simulink model "Simulation"  (R2024b)
settings: Solver=FixedStepAuto  StartTime=0.0  StopTime=inf  FixedStep=0.025  RelTol=1e-3
model workspace (MAT data in the model file):
  Ix = 1
  Ixy = 0
  Ixz = 0
  Iy = 1
  Iyx = 0
  Iyz = 0
  Iz = 1
  Izx = 0
  Izy = 0
  Kpd = 0
  Kqd = 0
  Krd = 0
  Kud = 0
  Kvd = 0
  Kwd = 0
  Mpd = 0
  Mqd = 0
  Mrd = 0
  Mud = 0
  Mvd = 0
  Mwd = 0
  Npd = 0
  Nqd = 0
  Nrd = 0
  Nud = 0
  Nvd = 0
  Nwd = 0
  Xpd = 0
  Xqd = 0
  Xrd = 0
  Xud = 0
  Xvd = 0
  Xwd = 0
  Ypd = 0
  Yqd = 0
  Yrd = 0
  Yud = 0
  Yvd = 0
  Ywd = 0
  Zpd = 0
  Zqd = 0
  Zrd = 0
  Zud = 0
  Zvd = 0
  Zwd = 0
  m = 35
  xg = 0
  yg = 0
  zg = 0
values from neighbouring files (symbols this model uses):
  force_values = force_values * 9.81    [initialize_data.m]    (also in matlab.mat = [-22.6611 -28.449 -34.5312 -39.9267 -45.0279 -49.4424 -22.56; vars.mat = [-22.6611 -28.449 -34.5312 -39.9267 -45.0279 -49.4424 -22.56)
  g = 9.81    [matlab.mat]    (also in vars.mat)
  pwm_values = unique(data(:, 2))    [initialize_data.m]    (also in matlab.mat = [1100 1104 1108 1112 1116 1120 1124 1128 1132 1136 1140 1144; vars.mat = [1100 1104 1108 1112 1116 1120 1124 1128 1132 1136 1140 1144)
  rho = 1000    [matlab.mat]
  thruster_dir = [0.5 0 0 0.5 0.5 0 0 0.5 -0.5 0 0 -0.5 ... (24 elements, 8x3)]    [matlab.mat]    (also in vars.mat)
  thruster_pos = [0.218 -0.218 -0.218 0.218 0.36 -0.36 -0.36 0.36 0.25 0.25 -0.25 -0.25 ... (24 elements, 8x3)]    [matlab.mat]    (also in vars.mat)
  V = 0.05061242    [matlab.mat]
  voltage_values = unique(data(:, 1))    [initialize_data.m]    (also in matlab.mat = [10 12 14 16 18 20]; vars.mat = [10 12 14 16 18 20])
libraries: sim3dlib x3, mssSimulink x1, ros2lib x1
settings Model: Creator=elite  LastModifiedBy=user

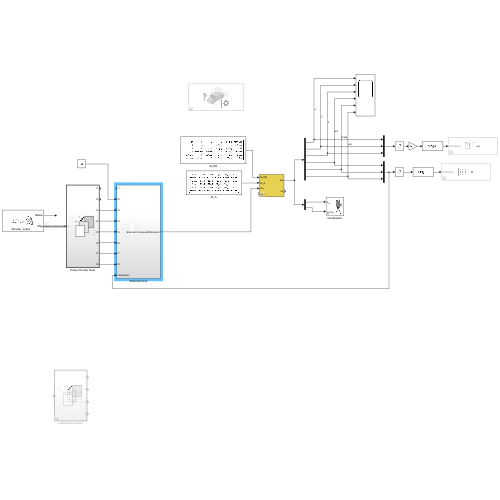
[thumbnail: Simulink's stored preview of the top-level diagram]
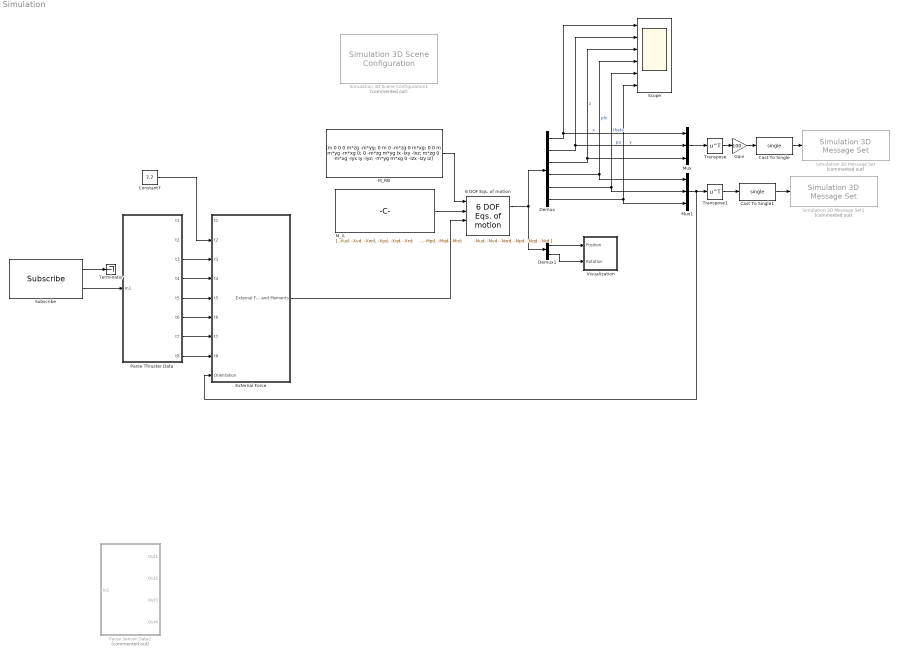
== system Simulation ==
  6 DOF Eqs. of motion : mssSimulink/Modelling/Kinetics /6 DOF Eqs. of motion  CoriolisOnOff=on  nu0=[0 0 0 0 0 0]  eta0=[0 0 0 0 0 0]
  Cast To Single : DataTypeConversion  OutDataTypeStr=single  SaturateOnIntegerOverflow=off  RndMeth=Floor
  Cast To Single1 : DataTypeConversion  OutDataTypeStr=single  SaturateOnIntegerOverflow=off  RndMeth=Floor
  Constant7 : Constant  Value=7.7
  Demux : Demux  Outputs=6
  Demux1 : Demux  Outputs=2
  External Force : Subsystem
  Gain : Gain  Gain=100
  M_A : Constant  Value=|  VectorParams1D=off
      | [ -Xud, -Xvd, -Xwd, -Xpd, -Xqd, -Xrd;
      |         -Yud, -Yvd, -Ywd, -Ypd, -Yqd, -Yrd;
      |         -Zud, -Zvd, -Zwd, -Zpd, -Zqd, -Zrd;
      |         -Kud, -Kvd, -Kwd, -Kpd, -Kqd, -Krd;
      |         -Mud, -Mvd, -Mwd, -Mpd, -Mqd, -Mrd;
      |         -Nud, -Nvd, -Nwd, -Npd, -Nqd, -Nrd ]
  M_RB : Constant  Value=|  VectorParams1D=off
      | [m 0 0 0 m*zg -m*yg; 
      |  0 m 0 -m*zg 0 m*xg; 
      |  0 0 m m*yg -m*xg 0; 
      |  0 -m*zg m*yg Ix -Ixy -Ixz; 
      |  m*zg 0 -m*xg -Iyx Iy -Iyz; 
      |  -m*yg m*xg 0 -Izx -Izy Iz]
  Mux : Mux  Inputs=3
  Mux1 : Mux  Inputs=3
  Parse Sensor Data1 : Subsystem  Commented=on  TreatAsAtomicUnit=on
  Parse Thruster Data : Subsystem  TreatAsAtomicUnit=on
  Scope : Scope  NumInputPorts=6
  Simulation 3D Message Set : sim3dlib/Simulation 3D Message Set  Priority=-1  Commented=on  SigName=pos  Ts=-1  aMode=2
      settings: LibrarySourceBlock=vehdynlibsim3dcore/Simulation 3D Message Set
  Simulation 3D Message Set1 : sim3dlib/Simulation 3D Message Set  Priority=-1  Commented=on  SigName=rot  Ts=-1  aMode=2
      settings: LibrarySourceBlock=vehdynlibsim3dcore/Simulation 3D Message Set
  Simulation 3D Scene Configuration1 : sim3dlib/Simulation 3D Scene Configuration  Priority=0  Commented=on  ProjectFormat=Unreal Editor  SceneDesc=Empty scene  ProjectName=C:\Program Files\MATLAB\R2024b\toolbox\shared\sim3d_projects\automotive_project_windows\UE\WindowsNoEditor\VehicleSimulation.exe  ScenePath=/Game/Maps/HwStrght  UEProjPath=C:\Users\user\Desktop\RoboSub MSDP\AUV_Visualization\AUV_Visualization.uproject  EnableOpenDRIVE=off  vehTagList={'Custom';'Scene Origin'}  vehTag=Scene Origin  FreeCameraInitialTranslation=[0, 0, 0]  FreeCameraDefaultInitialTranslation=[-6, 0, 2]  FreeCameraInitialRotation=[0, 0, 0]  FreeCameraDefaultInitialRotation=[0, -15, 0]  OpVisEn=off  Ts=0.025  EnableWindow=on  EnableRemoteAccess=off  EnableWeather=off  SunAzimuth=90  SunAltitude=40.0  EnableGeospatialSun=off  Latitude=0  Longitude=0  Date=2023-01-01  Time=10:30:00  GeoTimeZone=-5.0  SunDaylightSaving=off  wind=1  clouds=10  EnableVolumetricClouds=off  CloudCoverage=0  CloudAltitude=6  fog=0  rain=0  RaindropsEffect=off  SnowDensity=0  EnableGeospatial=off  UseTrueOrigin=off  OriginHeight=200  OriginLatitude=40.744652  OriginLongitude=-73.988864  MapStyle=Aerial  AdditionalAssetIDs=[]  UseAdvancedSunSky=off  SolarTime=11  TimeZone=-5  Day=21  Month=9  Year=2022  UseDaylightSavingTime=on  DSTStartDay=10  DSTStartMonth=3  DSTEndDay=3  DSTEndMonth=11  DSTSwitchHour=2  sensorTag=MainCamera2  sensorId=2  sensorName=MainCamera2  mountLoc=Origin  offsetFlag=off  tmountOffset=[0, 0, 0]  rmountOffset=[0, 0, 0]  HorizontalResolution=1280  VerticalResolution=720  HorizontalFOV=60  mountPoint=[0 0 0]  mountOrientation=[0 0 0]  aMode=5  ID=2  GeoTrigger=Inactive
      settings: LibrarySourceBlock=sl3dlib/Simulation 3D/Environment/Simulation 3D Scene Configuration
  Subscribe : ros2lib/Subscribe  topicSource=Select from ROS network  topic=/thruster_output  messageType=std_msgs/String  sampleTime=-1  QOSHistory=Keep last  QOSDepth=1  QOSReliability=Reliable  QOSDurability=Volatile  QOSDeadline=Inf  QOSLifespan=Inf  QOSLiveliness=Automatic  QOSLeaseDuration=Inf  QOSAvoidROSNamespaceConventions=off
  Terminator : Terminator
  Transpose : Math  Operator=transpose
  Transpose1 : Math  Operator=transpose
  Visualization : Subsystem  mask(6DoF_Animation){u2=0.1, u8=on}
      mask prompts: u2 "aeroblks:aeroblkanim6dof:block6DoF_AnimationParamTimeintervalbetweenupdates"; u8 "aeroblks:aeroblkanim6dof:block6DoF_AnimationParamEnableanimation"
      mask help: aeroblks:aeroblkanim6dof:block6DoF_AnimationDesc
      mask init:
      | aeroicon('aeroblk');
      | Config.update = u2;
      | Config.Animenable = u8;
      | Config.Model = bdroot(gcb);
      mask Help: eval('asbhelp(''sixdof_animation'')');
      mask DialogControl DescGroupVar Prompt: Animation
      mask DialogControl DescTextVar Prompt: Show animation of body
      mask DialogControl u2 Prompt: Time interval between updates:
      mask DialogControl u8 Prompt: Enable animation
      mask Display:
      | port_label('input',1,'x_e','texmode','on');
      | port_label('input',2,'\phi \theta \psi','texmode','on');
  wires:
  M_RB/1 -> 6 DOF Eqs. of motion/1
  M_A/1 -> 6 DOF Eqs. of motion/2
  6 DOF Eqs. of motion/1 -> Demux/1, Demux1/1
  Demux/1 -> Mux/1, Scope/1  "x"
  Demux/2 -> Mux/2, Scope/2  "y"
  Demux/4 -> Scope/4, Mux1/1  "phi"
  Demux/5 -> Scope/5, Mux1/2  "theta"
  Demux/6 -> Scope/6, Mux1/3  "psi"
  Demux/3 -> Mux/3, Scope/3  "z"
  Demux1/1 -> Visualization/1(Position)
  Demux1/2 -> Visualization/2(Rotation)
  Subscribe/2 -> Parse Thruster Data/1(In1)
  Subscribe/1 -> Terminator/1
  Mux1/1 -> External Force/9(Orientation), Transpose1/1
  Mux/1 -> Transpose/1
  Transpose/1 -> Gain/1
  Gain/1 -> Cast To Single/1
  Cast To Single/1 -> Simulation 3D Message Set/1
  Transpose1/1 -> Cast To Single1/1
  Cast To Single1/1 -> Simulation 3D Message Set1/1
  Constant7/1 -> External Force/2(t2)
  Parse Thruster Data/3(t3) -> External Force/3(t3)
  Parse Thruster Data/4(t4) -> External Force/4(t4)
  Parse Thruster Data/5(t5) -> External Force/5(t5)
  Parse Thruster Data/6(t6) -> External Force/6(t6)
  Parse Thruster Data/7(t7) -> External Force/7(t7)
  Parse Thruster Data/8(t8) -> External Force/8(t8)
  External Force/1(External Forces and Moments) -> 6 DOF Eqs. of motion/3

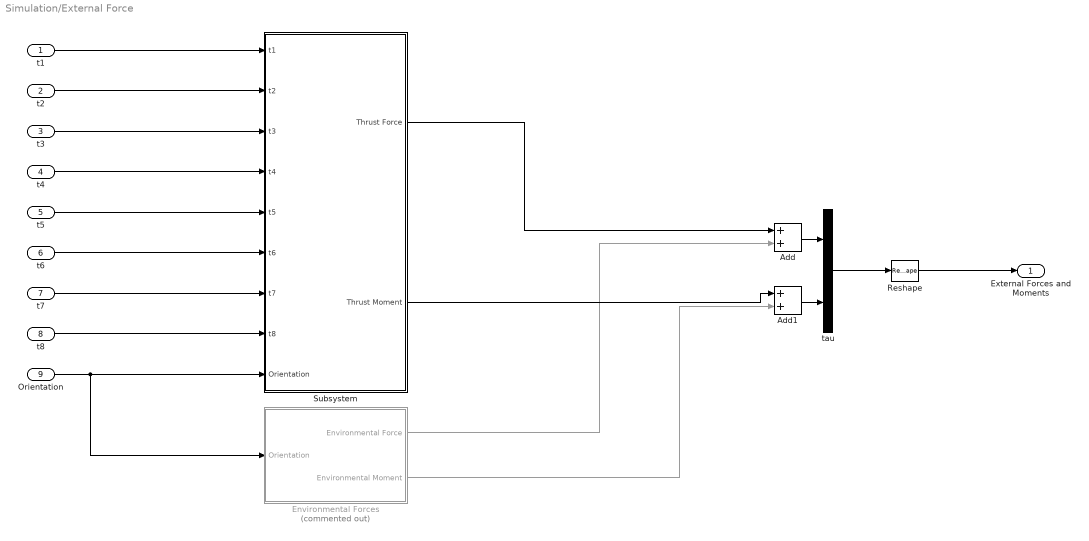
== system Simulation/External Force ==
  t1 : Inport
  t2 : Inport  Port=2
  t3 : Inport  Port=3
  t4 : Inport  Port=4
  t5 : Inport  Port=5
  t6 : Inport  Port=6
  t7 : Inport  Port=7
  t8 : Inport  Port=8
  Orientation : Inport  Port=9
  Add : Sum
  Add1 : Sum
  Environmental Forces : Subsystem  Commented=on
  Reshape : Reshape
  Subsystem : Subsystem
  tau : Mux  Inputs=2
  External Forces and Moments : Outport
  wires:
  tau/1 -> Reshape/1
  Reshape/1 -> External Forces and Moments/1
  Environmental Forces/1(Environmental Force) -> Add/2
  t1/1 -> Subsystem/1(t1)
  t2/1 -> Subsystem/2(t2)
  t3/1 -> Subsystem/3(t3)
  t4/1 -> Subsystem/4(t4)
  t5/1 -> Subsystem/5(t5)
  t6/1 -> Subsystem/6(t6)
  t7/1 -> Subsystem/7(t7)
  t8/1 -> Subsystem/8(t8)
  Orientation/1 -> Environmental Forces/1(Orientation), Subsystem/9(Orientation)
  Subsystem/1(Thrust Force) -> Add/1
  Add/1 -> tau/1
  Add1/1 -> tau/2
  Subsystem/2(Thrust Moment) -> Add1/1
  Environmental Forces/2(Environmental Moment) -> Add1/2

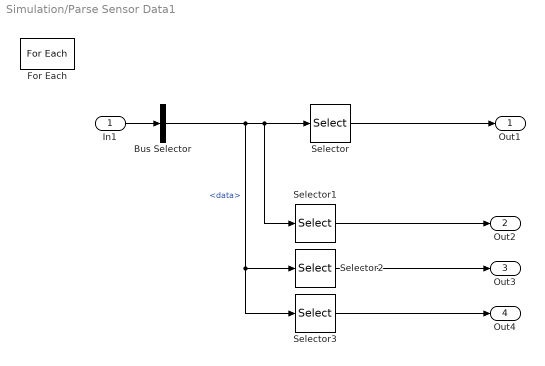
== system Simulation/Parse Sensor Data1 ==
  In1 : Inport  Partition=on  PartitionDimension=1  PartitionWidth=1  PartitionOffset=0
  Bus Selector : BusSelector  OutputSignals=data
  For Each : ForEach  DisableCoverage=on
  Selector : Selector  InputPortWidth=128  IndexOptions=Index vector (dialog)  Indices=1  OutputSizes=1
  Selector1 : Selector  InputPortWidth=128  IndexOptions=Index vector (dialog)  Indices=2  OutputSizes=1
  Selector2 : Selector  InputPortWidth=128  IndexOptions=Index vector (dialog)  Indices=3  OutputSizes=1
  Selector3 : Selector  InputPortWidth=128  IndexOptions=Index vector (dialog)  Indices=4  OutputSizes=1
  Out1 : Outport  ConcatenationDimension=1
  Out2 : Outport  Port=2  ConcatenationDimension=1
  Out3 : Outport  Port=3  ConcatenationDimension=1
  Out4 : Outport  Port=4  ConcatenationDimension=1
  wires:
  In1/1 -> Bus Selector/1
  Selector3/1 -> Out4/1
  Selector/1 -> Out1/1
  Selector2/1 -> Out3/1
  Selector1/1 -> Out2/1
  Bus Selector/1 -> Selector/1, Selector1/1, Selector3/1, Selector2/1  "<data>"

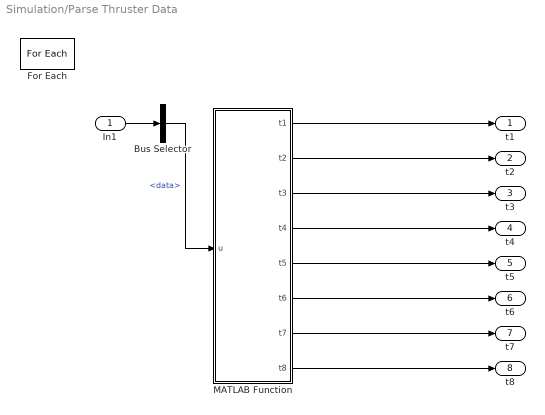
== system Simulation/Parse Thruster Data ==
  In1 : Inport  Partition=on  PartitionDimension=1  PartitionWidth=1  PartitionOffset=0
  Bus Selector : BusSelector  OutputSignals=data
  For Each : ForEach  DisableCoverage=on
  MATLAB Function : MATLAB Function  TreatAsAtomicUnit=on
  t1 : Outport  ConcatenationDimension=1
  t2 : Outport  Port=2  ConcatenationDimension=1
  t3 : Outport  Port=3  ConcatenationDimension=1
  t4 : Outport  Port=4  ConcatenationDimension=1
  t5 : Outport  Port=5  ConcatenationDimension=1
  t6 : Outport  Port=6  ConcatenationDimension=1
  t7 : Outport  Port=7  ConcatenationDimension=1
  t8 : Outport  Port=8  ConcatenationDimension=1
  wires:
  In1/1 -> Bus Selector/1
  MATLAB Function/4(t4) -> t4/1
  MATLAB Function/1(t1) -> t1/1
  MATLAB Function/3(t3) -> t3/1
  MATLAB Function/2(t2) -> t2/1
  Bus Selector/1 -> MATLAB Function/1(u)  "<data>"
  MATLAB Function/5(t5) -> t5/1
  MATLAB Function/6(t6) -> t6/1
  MATLAB Function/7(t7) -> t7/1
  MATLAB Function/8(t8) -> t8/1

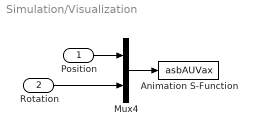
== system Simulation/Visualization ==
  Position : Inport
  Rotation : Inport  Port=2  Unit=rad
  Animation S-Function : M-S-Function  FunctionName=asbAUVax  Parameters=Config
  Mux4 : Mux  Inputs=2
  wires:
  Rotation/1 -> Mux4/2
  Mux4/1 -> Animation S-Function/1
  Position/1 -> Mux4/1

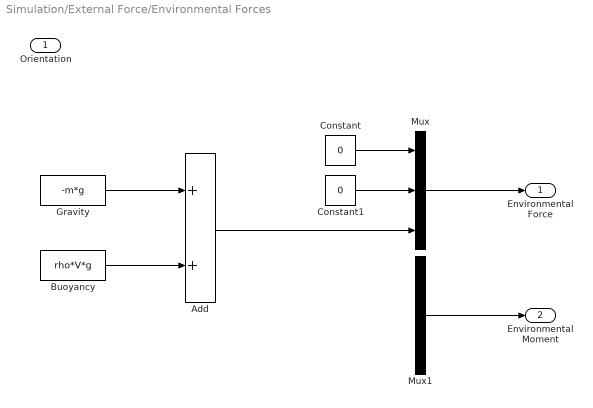
== system Simulation/External Force/Environmental Forces ==
  Orientation : Inport
  Add : Sum
  Buoyancy : Constant  Value=rho*V*g
  Constant : Constant  Value=0
  Constant1 : Constant  Value=0
  Gravity : Constant  Value=-m*g
  Mux : Mux  Inputs=3
  Mux1 : Mux  Inputs=3
  Environmental Force : Outport
  Environmental Moment : Outport  Port=2
  wires:
  Buoyancy/1 -> Add/2
  Gravity/1 -> Add/1
  Mux/1 -> Environmental Force/1
  Add/1 -> Mux/3
  Constant/1 -> Mux/1
  Constant1/1 -> Mux/2
  Mux1/1 -> Environmental Moment/1

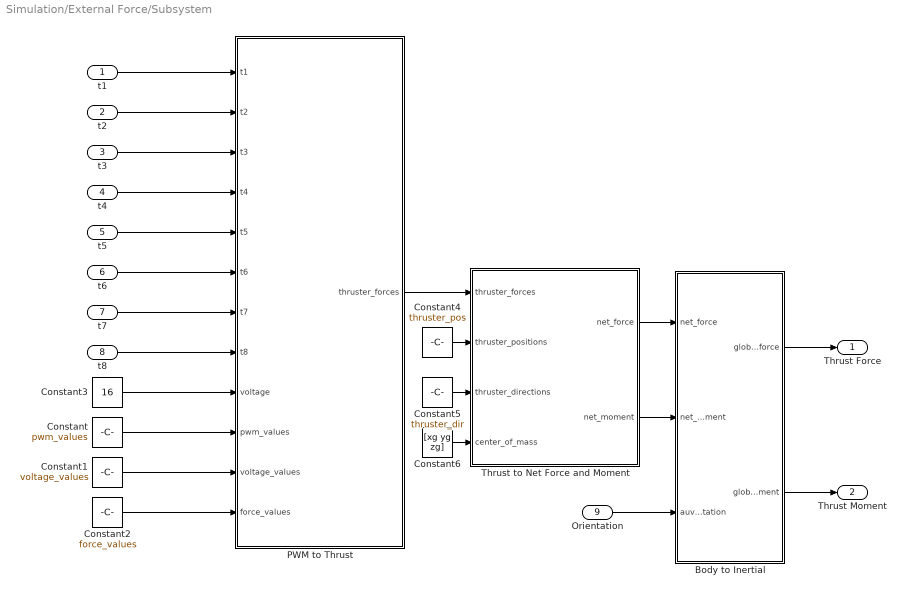
== system Simulation/External Force/Subsystem ==
  t1 : Inport
  t2 : Inport  Port=2
  t3 : Inport  Port=3
  t4 : Inport  Port=4
  t5 : Inport  Port=5
  t6 : Inport  Port=6
  t7 : Inport  Port=7
  t8 : Inport  Port=8
  Orientation : Inport  Port=9
  Body to Inertial : MATLAB Function  TreatAsAtomicUnit=on
  Constant : Constant  Value=pwm_values
  Constant1 : Constant  Value=voltage_values
  Constant2 : Constant  Value=force_values
  Constant3 : Constant  Value=16
  Constant4 : Constant  Value=thruster_pos
  Constant5 : Constant  Value=thruster_dir
  Constant6 : Constant  Value=[xg yg zg]  VectorParams1D=off
  PWM to Thrust : MATLAB Function  TreatAsAtomicUnit=on
  Thrust to Net Force and Moment : MATLAB Function  TreatAsAtomicUnit=on
  Thrust Force : Outport
  Thrust Moment : Outport  Port=2
  wires:
  Thrust to Net Force and Moment/2(net_moment) -> Body to Inertial/2(net_moment)
  Constant2/1 -> PWM to Thrust/12(force_values)
  Constant1/1 -> PWM to Thrust/11(voltage_values)
  Constant5/1 -> Thrust to Net Force and Moment/3(thruster_directions)
  t1/1 -> PWM to Thrust/1(t1)
  PWM to Thrust/1(thruster_forces) -> Thrust to Net Force and Moment/1(thruster_forces)
  Constant6/1 -> Thrust to Net Force and Moment/4(center_of_mass)
  Constant4/1 -> Thrust to Net Force and Moment/2(thruster_positions)
  Constant/1 -> PWM to Thrust/10(pwm_values)
  Constant3/1 -> PWM to Thrust/9(voltage)
  Thrust to Net Force and Moment/1(net_force) -> Body to Inertial/1(net_force)
  t4/1 -> PWM to Thrust/4(t4)
  t5/1 -> PWM to Thrust/5(t5)
  Body to Inertial/1(global_force) -> Thrust Force/1
  t6/1 -> PWM to Thrust/6(t6)
  t7/1 -> PWM to Thrust/7(t7)
  t8/1 -> PWM to Thrust/8(t8)
  Orientation/1 -> Body to Inertial/3(auv_orientation)
  t2/1 -> PWM to Thrust/2(t2)
  t3/1 -> PWM to Thrust/3(t3)
  Body to Inertial/2(global_moment) -> Thrust Moment/1

== matlab function Simulation/External Force/Subsystem/PWM to Thrust ==
  data: t1 input; thruster_forces output; t2 input; t3 input; t4 input; t5 input; t6 input; t7 input; t8 input; voltage input; pwm_values input; voltage_values input; force_values input
function thruster_forces = dutyCycleToThrusterForces(t1, t2, t3, t4, t5, t6, t7, t8, voltage, pwm_values, voltage_values, force_values)
    % Define min/max values for duty cycle and PWM
    duty_min = 5.5;
    duty_max = 9.5;
    pwm_min = 1100;
    pwm_max = 1900;

    % Create an array for the input duty cycles
    vals = [t1, t2, t3, t4, t5, t6, t7, t8];
    duty_cycle_array = arrayfun(@(x) 7.5 * (isempty(x) || x == 0 || isnan(x)) + x * ~(isempty(x) || x == 0 || isnan(x)), vals);

    % Convert duty cycle to PWM using linear scaling
    pwm_array = pwm_min + ((duty_cycle_array - duty_min) / (duty_max - duty_min)) * (pwm_max - pwm_min);

    % Clip PWM values to the valid range (1100 - 1900)
    pwm_array = min(max(pwm_array, pwm_min), pwm_max);

    % Interpolate forces for each PWM value at the given voltage
    thruster_forces = zeros(1, 8);  % Initialize output array
    for idx = 1:length(pwm_array)
        % Interpolate using 2D interpolation (PWM and voltage)
        thruster_forces(idx) = interp2(pwm_values, voltage_values, force_values, pwm_array(idx), voltage, 'linear');
    end
end

== matlab function Simulation/Parse Thruster Data/MATLAB Function ==
  data: u input; t1 output; t2 output; t3 output; t4 output; t5 output; t6 output; t7 output; t8 output
function [t1, t2, t3, t4, t5, t6, t7, t8] = fcn(u)
    % This function splits the input string 'u' into 8 separate variables (t1 to t8)
    u = char(u); % Ensure that the input is in char array format
    
    % Initialize an array to hold the split values
    split_values = zeros(1, 8);
    
    % Convert input string to a character array (e.g., '7.5,7.5,7.5,7.5,7.5,7.5,7.5,7.5')
    idx = 1; % Index for the split values
    startIdx = 1; % Start index for each value
    
    for i = 1:length(u)
        % Check if we encounter a comma, which separates the values
        if u(i) == ',' || i == length(u)
            % Extract the number before the comma (or the last value in the string)
            if i == length(u)
                temp_val = str2double(u(startIdx:end)); % Last value
            else
                temp_val = str2double(u(startIdx:i-1)); % Value before comma
            end
            
            % Ensure the conversion is successful (not NaN)
            if ~isnan(temp_val)
                split_values(idx) = real(temp_val); % Assign the real part if valid
            else
                error('Invalid number format in input string at position %d.', idx);
            end
            
            idx = idx + 1; % Move to the next index
            startIdx = i + 1; % Update the start index for the next value
        end
    end
    
    % Ensure that the input string contains exactly 8 values
    if idx - 1 ~= 8
        error('The input string must contain exactly 8 numeric values.');
    end
    
    % Assign each value to the corresponding output variable
    t1 = split_values(1);
    t2 = split_values(2);
    t3 = split_values(3);
    t4 = split_values(4);
    t5 = split_values(5);
    t6 = split_values(6);
    t7 = split_values(7);
    t8 = split_values(8);
end

== matlab function Simulation/External Force/Subsystem/Thrust to Net Force and Moment ==
  data: thruster_forces input; thruster_positions input; net_force output; thruster_directions input; center_of_mass input; net_moment output
function [net_force, net_moment] = computeNetForceAndMoment(thruster_forces, thruster_positions, thruster_directions, center_of_mass)
    % Computes the net force and net moment on the AUV given the positions, forces, and directions of thrusters
    %
    % Parameters:
    % thruster_positions: Nx3 matrix of thruster positions [x, y, z]
    % thruster_forces: Nx1 vector of force magnitudes for each thruster
    % thruster_directions: Nx3 matrix of thruster directions [dx, dy, dz]
    % center_of_mass: 1x3 vector representing the AUV's center of mass [x, y, z]
    %
    % Returns:
    % net_force: 1x3 vector representing the net force on the AUV [Fx, Fy, Fz]
    % net_moment: 1x3 vector representing the net moment on the AUV [Mx, My, Mz]

    num_thrusters = size(thruster_positions, 1);  % Number of thrusters

    % Initialize net force and net moment to zero
    f = [0, 0, 0];  % [Fx, Fy, Fz]
    m = [0, 0, 0];  % [Mx, My, Mz]

    % Iterate through each thruster to calculate force components and moments
    for i = 1:num_thrusters
        % Extract the direction vector
        direction_vector = thruster_directions(i, :);
        
        % Normalize the direction vector
        normalized_vector = direction_vector / norm(direction_vector);
        
        % Compute the force vector by scaling with the force magnitude
        force_vector = thruster_forces(i) * normalized_vector;
        
        % Accumulate net force
        f = f + force_vector;
        
        % Compute the position vector relative to the center of mass
        position_relative_to_com = thruster_positions(i, :) - center_of_mass;
        
        % Calculate the moment generated by the thruster using the cross product
        moment_vector = cross(position_relative_to_com, force_vector);
        
        % Accumulate net moment
        m = m + moment_vector;
    end

    % Ensure net_force and net_moment are column vectors
    net_force = f(:); 
    net_moment = m(:);
end

== matlab function Simulation/External Force/Subsystem/Body to Inertial ==
  data: net_force input; global_force output; net_moment input; auv_orientation input; global_moment output
function [global_force, global_moment] = convertToGlobal(net_force, net_moment, auv_orientation)
    % Convert orientation angles from degrees to radians
    pitch = deg2rad(auv_orientation(1)); 
    roll  = deg2rad(auv_orientation(2)); 
    yaw   = deg2rad(auv_orientation(3)); 

    % Rotation Matrices
    R_x = [1, 0, 0;
           0, cos(pitch), -sin(pitch);
           0, sin(pitch), cos(pitch)];
       
    R_y = [cos(roll), 0, sin(roll);
           0, 1, 0;
          -sin(roll), 0, cos(roll)];
      
    R_z = [cos(yaw), -sin(yaw), 0;
           sin(yaw), cos(yaw), 0;
           0, 0, 1];

    % Full Rotation Matrix (Global to AUV Frame)
    R = R_z * R_y * R_x; 

    % Convert forces and moments to the global frame
    global_force = R * net_force;
    %global_force = global_force(:);
    global_moment = R * net_moment;
    %global_moment = global_moment(:);
end
